simulink model "Cruise_Control_plant_model_with_continuous_controller"  (R2026a)
settings: Solver=VariableStepAuto  StopTime=inf
model workspace (MAT data in the model file):
  Crr = 0.015
  DragCoeff = 50
  MaxBrakeForce_N = 8000
  MaxEngineForce_N = 4000
  MaxVehicleSpeed_mps = 50
  MinCruiseSpd = 20
  Vehicle_mass_kg = 1000
  g = 9.81
libraries: slpidlib x1
settings Model: Creator=irfan  LastModifiedBy=irfan

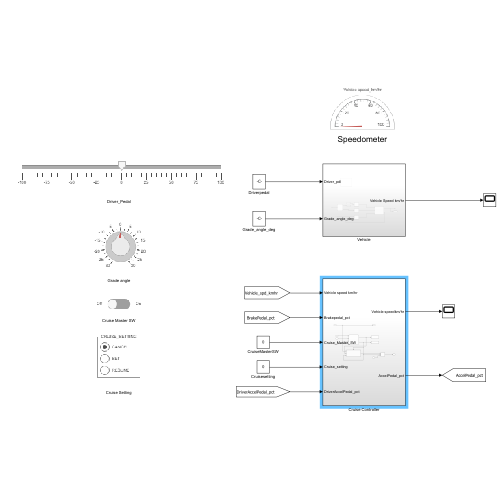
[thumbnail: Simulink's stored preview of the top-level diagram]
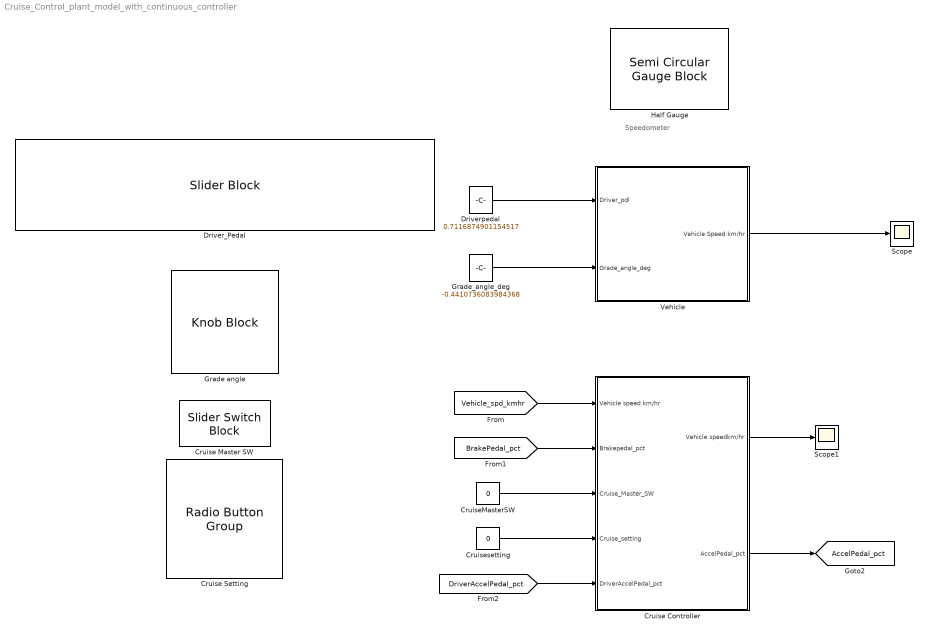
== system Cruise_Control_plant_model_with_continuous_controller ==
  note: Speedometer
  Cruise Controller : Subsystem
  Cruise Master SW : SliderSwitchBlock  LabelPosition=Hide
  Cruise Setting : RadioButtonGroup  LabelPosition=Hide  SelectedLabel=CANCEL  ButtonGroupName=CRUISE_SETTING
  CruiseMasterSW : Constant  Value=0
  Cruisesetting : Constant  Value=0
  Driver_Pedal : SliderBlock  LabelPosition=Hide  ScaleMin=-100  TickInterval=25
  Driverpedal : Constant  Value=0.7116874901154517
  Grade angle : KnobBlock  LabelPosition=Hide  ScaleMin=-30  ScaleMax=30  TickInterval=5
  Grade_angle_deg : Constant  Value=-0.4410736083984368
  Half Gauge : SemiCircularGaugeBlock  FontColor=[0.0, 0.0, 0.0]
  Scope : Scope
      settings: ActiveDisplayYMinimum=-1  ActiveDisplayYMaximum=1
  Scope1 : Scope
      settings: ActiveDisplayYMinimum=-1  ActiveDisplayYMaximum=1
  Vehicle : Subsystem
  tag scope: AccelPedal_pct=global
  wires:
  Vehicle/1(Vehicle Speed km/hr) -> Scope/1
  Driverpedal/1 -> Vehicle/1(Driver_pdl)
  Grade_angle_deg/1 -> Vehicle/2(Grade_angle_deg)
  [Vehicle_spd_kmhr] -> Cruise Controller/1(Vehicle speed km/hr)
  [BrakePedal_pct] -> Cruise Controller/2(Brakepedal_pct)
  Cruisesetting/1 -> Cruise Controller/4(Cruise_setting)
  CruiseMasterSW/1 -> Cruise Controller/3(Cruise_Master_SW)
  [DriverAccelPedal_pct] -> Cruise Controller/5(DriverAccelPedal_pct)
  Cruise Controller/2(AccelPedal_pct) -> [AccelPedal_pct]
  Cruise Controller/1(Vehicle speedkm/hr) -> Scope1/1

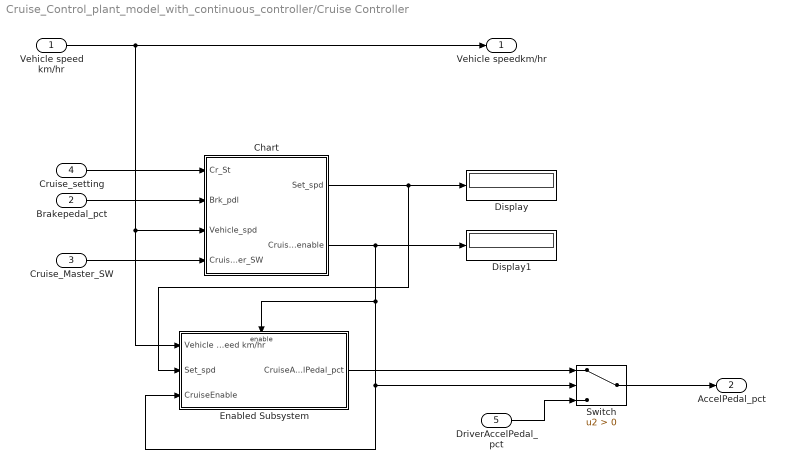
== system Cruise_Control_plant_model_with_continuous_controller/Cruise Controller ==
  Vehicle speed km/hr : Inport
  Brakepedal_pct : Inport  Port=2
  Cruise_Master_SW : Inport  Port=3
  Cruise_setting : Inport  Port=4
  DriverAccelPedal_pct : Inport  Port=5
  Chart : Stateflow chart  TreatAsAtomicUnit=on
  Display : Display
  Display1 : Display
  Enabled Subsystem : Subsystem  TreatAsAtomicUnit=on
  Switch : Switch  Criteria=u2 > Threshold  SaturateOnIntegerOverflow=off  InputSameDT=off
  Vehicle speedkm/hr : Outport
  AccelPedal_pct : Outport  Port=2
  wires:
  Cruise_setting/1 -> Chart/1(Cr_St)
  Brakepedal_pct/1 -> Chart/2(Brk_pdl)
  Vehicle speed km/hr/1 -> Vehicle speedkm/hr/1, Chart/3(Vehicle_spd), Enabled Subsystem/1(Vehicle speed km/hr)
  Chart/1(Set_spd) -> Enabled Subsystem/2(Set_spd), Display/1
  Chart/2(Cruise_enable) -> Display1/1, Enabled Subsystem/Enable, Enabled Subsystem/3(CruiseEnable), Switch/2
  Cruise_Master_SW/1 -> Chart/4(Cruise_Master_SW)
  Enabled Subsystem/1(CruiseAccelPedal_pct) -> Switch/1
  DriverAccelPedal_pct/1 -> Switch/3
  Switch/1 -> AccelPedal_pct/1

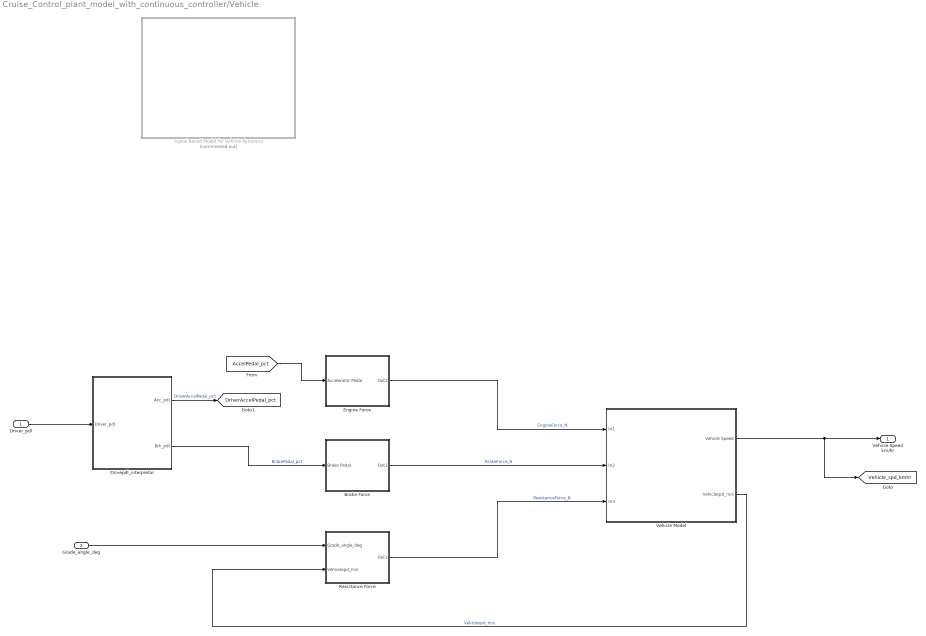
== system Cruise_Control_plant_model_with_continuous_controller/Vehicle ==
  Driver_pdl : Inport
  Grade_angle_deg : Inport  Port=2
  Brake Force : Subsystem
  Drivepdl_interpretor : Subsystem
  Engine Force : Subsystem
  Resistance Force : Subsystem
  Signal Based Model for Vehicle dynamics : Subsystem  Commented=on
  Vehicle Model : Subsystem
  Vehicle Speed km/hr : Outport
  tag scope: DriverAccelPedal_pct=global, Vehicle_spd_kmhr=global
  wires:
  Engine Force/1(Out1) -> Vehicle Model/1(In1)  "EngineForce_N"
  Brake Force/1(Out1) -> Vehicle Model/2(In2)  "BrakeForce_N"
  Drivepdl_interpretor/2(Brk_pdl) -> Brake Force/1(Brake Pedal)  "BrakePedal_pct"
  Resistance Force/1(Out1) -> Vehicle Model/3(In3)  "ResistanceForce_N"
  Vehicle Model/2(Vehiclespd_m/s) -> Resistance Force/2(Vehiclespd_m/s)  "Vehiclespd_m/s"
  Vehicle Model/1(Vehicle Speed) -> [Vehicle_spd_kmhr], Vehicle Speed km/hr/1
  Driver_pdl/1 -> Drivepdl_interpretor/1(Driver_pdl)
  Grade_angle_deg/1 -> Resistance Force/1(Grade_angle_deg)
  Drivepdl_interpretor/1(Acc_pdl) -> [DriverAccelPedal_pct]  "DriverAccelPedal_pct"
  [AccelPedal_pct] -> Engine Force/1(Accelerator Pedal)

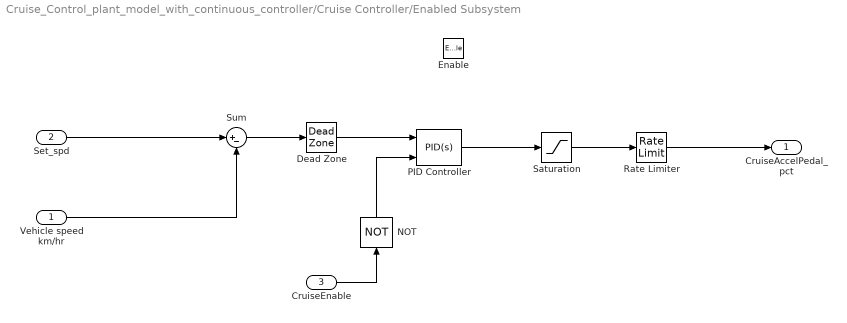
== system Cruise_Control_plant_model_with_continuous_controller/Cruise Controller/Enabled Subsystem ==
  Vehicle speed km/hr : Inport
  Set_spd : Inport  Port=2
  CruiseEnable : Inport  Port=3
  Enable : EnablePort  StatesWhenEnabling=reset
  Dead Zone : DeadZone
  NOT : Logic  Operator=NOT  IconShape=distinctive  AllPortsSameDT=off  OutDataTypeStr=boolean
  PID Controller : slpidlib/PID Controller  Controller=PID  Form=Parallel  TimeDomain=Continuous-time  UseExternalTs=off  SampleTime=-1  IntegratorMethod=Forward Euler  FilterMethod=Forward Euler  ControllerParametersSource=internal  P=1  I=0.5  UseKiTs=off  D=0  UseExternalDerivativeSource=off  N=100  UseFilter=on  TunerSelectOption=Transfer Function Based (PID Tuner App)  InitialConditionSource=internal  InitialConditionForIntegrator=0  InitialConditionForFilter=0  DifferentiatorICPrevScaledInput=0  ExternalReset=rising  TrackingMode=off  Kt=1  LimitOutput=on  SatLimitsSource=internal  UpperSaturationLimit=100  LowerSaturationLimit=0  LinearizeAsGain=on  AntiWindupMode=back-calculation  Kb=1  LimitIntegrator=off  UpperIntegratorSaturationLimit=inf  LowerIntegratorSaturationLimit=-inf  POutMin=[]  POutMax=[]  IOutMin=[]  IOutMax=[]  DOutMin=[]  DOutMax=[]  NOutMin=[]  NOutMax=[]  SumOutMin=[]  SumOutMax=[]  SaturationOutMin=[]  SaturationOutMax=[]  PParamMin=[]  PParamMax=[]  IParamMin=[]  IParamMax=[]  DParamMin=[]  DParamMax=[]  NParamMin=[]  NParamMax=[]  KbParamMin=[]  KbParamMax=[]  KtParamMin=[]  KtParamMax=[]  KbOutMin=[]  KbOutMax=[]  KtOutMin=[]  KtOutMax=[]  IntegratorOutMin=[]  IntegratorOutMax=[]  FilterOutMin=[]  FilterOutMax=[]  SumI1OutMin=[]  SumI1OutMax=[]  SumI2OutMin=[]  SumI2OutMax=[]  SumI3OutMin=[]  SumI3OutMax=[]  SumI4OutMin=[]  SumI4OutMax=[]  SumDOutMin=[]  SumDOutMax=[]  DifferentiatorOutMin=[]  DifferentiatorOutMax=[]  FilterDiffOutCoefMin=[]  FilterDiffOutCoefMax=[]  ReciprocalOutMin=[]  ReciprocalOutMax=[]  SumDenOutMin=[]  SumDenOutMax=[]  SumNumOutMin=[]  SumNumOutMax=[]  DivideOutMin=[]  DivideOutMax=[]  UdiffTsProdOutMin=[]  UdiffTsProdOutMax=[]  NTsProdOutMin=[]  NTsProdOutMax=[]  UintegralTsProdOutMin=[]  UintegralTsProdOutMax=[]  UngainTsProdOutMin=[]  UngainTsProdOutMax=[]  ClampingZeroOutDataTypeStr=Inherit: Inherit via back propagation  ClampingZeroOutMin=[]  ClampingZeroOutMax=[]  FilterDenConstantOutDataTypeStr=Inherit: Inherit via back propagation  FilterDenConstantOutMin=[]  FilterDenConstantOutMax=[]  PCopyOutDataTypeStr=Inherit: Inherit via back propagation  PCopyOutMin=[]  PCopyOutMax=[]  NCopyOutDataTypeStr=Inherit: Inherit via back propagation  NCopyOutMin=[]  NCopyOutMax=[]  IntegratorContinuousStateAttributes=''  IntegratorStateMustResolveToSignalObject=off  IntegratorRTWStateStorageClass=Auto  FilterContinuousStateAttributes=''  FilterStateMustResolveToSignalObject=off  FilterRTWStateStorageClass=Auto  ParallelPVariant=InternalParameters  IdealPVariant=Disabled  IVariant=InternalParameters  DVariant=InternalParameters  IntegratorVariant=Continuous  SatVariant=Enabled  AWVariant=BackCalculation  PCopyVariant=Disabled  TRVariant=Disabled  FdbkBlocksVariant=Forward  IdealPFdbkVariant=Disabled  SatFdbkVariant=Disabled  DerivativeFilterVariant=ContFilter  NVariant=InternalParameters  NCopyVariant=Disabled  FilterICVariant=InternalICsFilter  IntegratorICVariant=InternalICs  ExternalResetVariant=ExternalReset  TRSumVariant=Passthrough  SumFdbkVariant=Disabled  SumVariant=Sum_PID  TsampFilterVariant=InternalTs  TsampNgainVariant=Passthrough  TsampIntegralVariant=Disabled_SignalSpec  ExternalSaturationOutDataTypeStr=Inherit: Same as second input  DerivativeSourceVariant=ErrorSignal  PreIntVariant=InternalPreInt
  Rate Limiter : RateLimiter  RisingSlewLimit=25  FallingSlewLimit=-40  SampleTimeMode=inherited
  Saturation : Saturate  UpperLimit=100  LowerLimit=0
  Sum : Sum  Inputs=|+-
  CruiseAccelPedal_pct : Outport
  wires:
  Sum/1 -> Dead Zone/1
  Saturation/1 -> Rate Limiter/1
  CruiseEnable/1 -> NOT/1
  NOT/1 -> PID Controller/2
  Vehicle speed km/hr/1 -> Sum/2
  Set_spd/1 -> Sum/1
  PID Controller/1 -> Saturation/1
  Rate Limiter/1 -> CruiseAccelPedal_pct/1
  Dead Zone/1 -> PID Controller/1

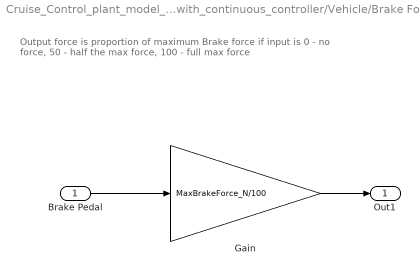
== system Cruise_Control_plant_model_with_continuous_controller/Vehicle/Brake Force ==
  note: Output force is proportion of maximum Brake force
      | if input is 0 - no force, 50 - half the max force, 100 - full max force
  Brake Pedal : Inport
  Gain : Gain  Gain=MaxBrakeForce_N/100
  Out1 : Outport
  wires:
  Brake Pedal/1 -> Gain/1
  Gain/1 -> Out1/1

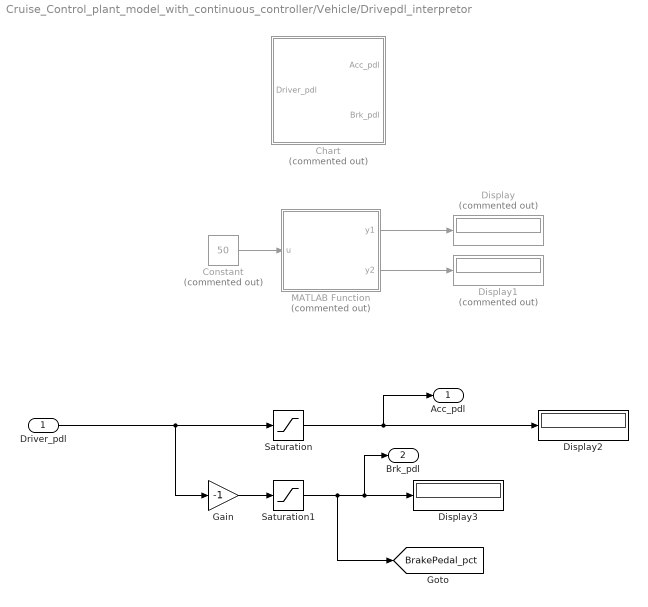
== system Cruise_Control_plant_model_with_continuous_controller/Vehicle/Drivepdl_interpretor ==
  Driver_pdl : Inport
  Chart : Stateflow chart  Commented=on  TreatAsAtomicUnit=on
  Constant : Constant  Commented=on  Value=50
  Display : Display  Commented=on
  Display1 : Display  Commented=on
  Display2 : Display
  Display3 : Display
  Gain : Gain  Gain=-1
  MATLAB Function : MATLAB Function  Commented=on  TreatAsAtomicUnit=on
  Saturation : Saturate  UpperLimit=100  LowerLimit=0
  Saturation1 : Saturate  UpperLimit=100  LowerLimit=0
  Acc_pdl : Outport
  Brk_pdl : Outport  Port=2
  tag scope: BrakePedal_pct=global
  wires:
  Constant/1 -> MATLAB Function/1(u)
  MATLAB Function/1(y1) -> Display/1
  MATLAB Function/2(y2) -> Display1/1
  Driver_pdl/1 -> Gain/1, Saturation/1
  Saturation/1 -> Acc_pdl/1, Display2/1
  Saturation1/1 -> [BrakePedal_pct], Brk_pdl/1, Display3/1
  Gain/1 -> Saturation1/1

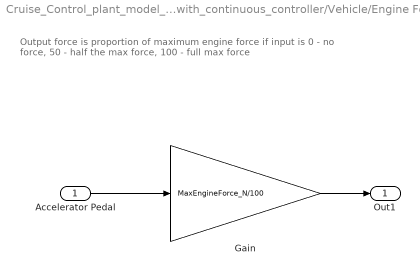
== system Cruise_Control_plant_model_with_continuous_controller/Vehicle/Engine Force ==
  note: Output force is proportion of maximum engine force
      | if input is 0 - no force, 50 - half the max force, 100 - full max force
  Accelerator Pedal : Inport
  Gain : Gain  Gain=MaxEngineForce_N/100
  Out1 : Outport
  wires:
  Accelerator Pedal/1 -> Gain/1
  Gain/1 -> Out1/1

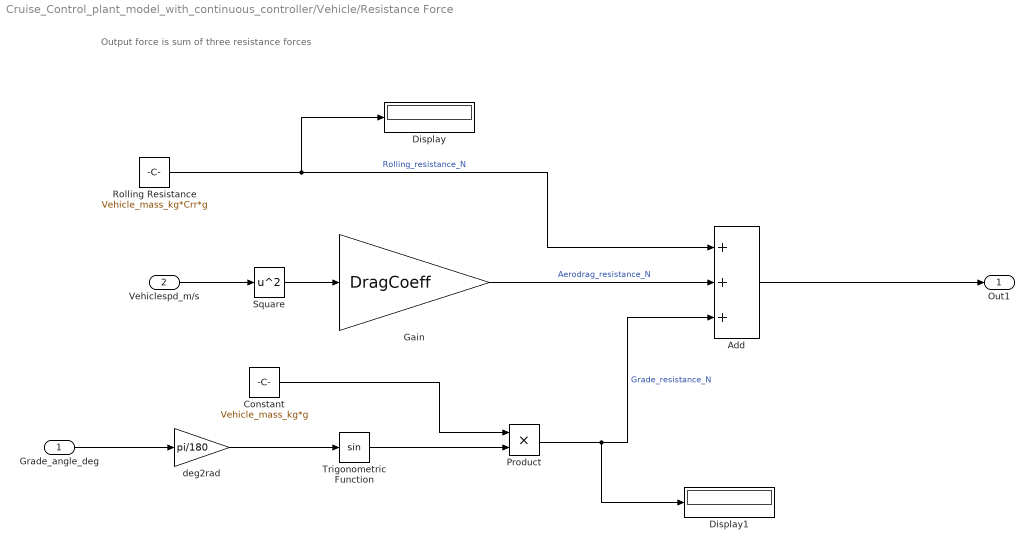
== system Cruise_Control_plant_model_with_continuous_controller/Vehicle/Resistance Force ==
  note: Output force is sum of three resistance forces
  Grade_angle_deg : Inport
  Vehiclespd_m/s : Inport  Port=2
  Add : Sum  Inputs=+++
  Constant : Constant  Value=Vehicle_mass_kg*g
  Display : Display
  Display1 : Display
  Gain : Gain  Gain=DragCoeff
  Product : Product
  Rolling Resistance : Constant  Value=Vehicle_mass_kg*Crr*g
  Square : Math  Operator=square
  Trigonometric Function : Trigonometry
  deg2rad : Gain  Gain=pi/180
  Out1 : Outport
  wires:
  Vehiclespd_m/s/1 -> Square/1
  Gain/1 -> Add/2  "Aerodrag_resistance_N"
  Rolling Resistance/1 -> Display/1, Add/1  "Rolling_resistance_N"
  Square/1 -> Gain/1
  Add/1 -> Out1/1
  Grade_angle_deg/1 -> deg2rad/1
  deg2rad/1 -> Trigonometric Function/1
  Trigonometric Function/1 -> Product/2
  Constant/1 -> Product/1
  Product/1 -> Display1/1, Add/3  "Grade_resistance_N"

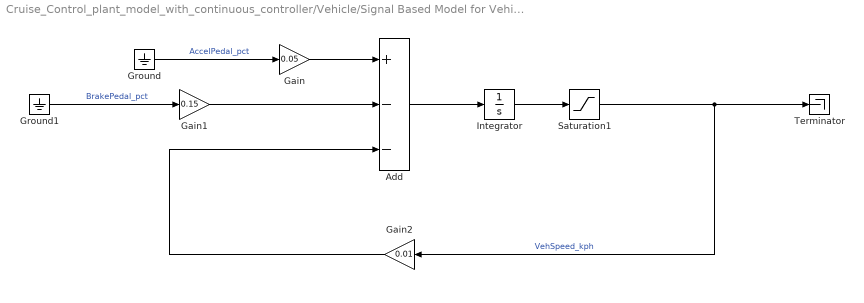
== system Cruise_Control_plant_model_with_continuous_controller/Vehicle/Signal Based Model for Vehicle dynamics ==
  Add : Sum  Inputs=+--
  Gain : Gain  Gain=0.05
  Gain1 : Gain  Gain=0.15
  Gain2 : Gain  Gain=0.01
  Ground : Ground
  Ground1 : Ground
  Integrator : Integrator
  Saturation1 : Saturate  UpperLimit=180  LowerLimit=0
  Terminator : Terminator
  wires:
  Ground1/1 -> Gain1/1  "BrakePedal_pct"
  Add/1 -> Integrator/1
  Gain/1 -> Add/1
  Gain2/1 -> Add/3
  Gain1/1 -> Add/2
  Saturation1/1 -> Terminator/1, Gain2/1  "VehSpeed_kph"
  Ground/1 -> Gain/1  "AccelPedal_pct"
  Integrator/1 -> Saturation1/1

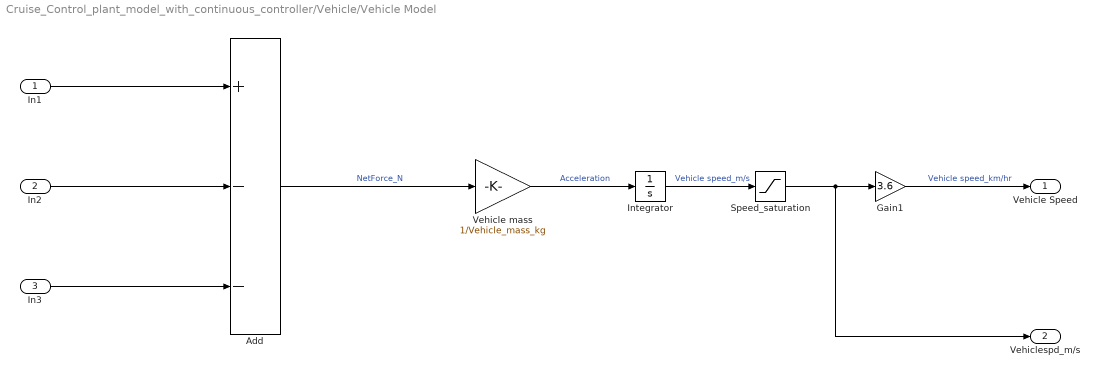
== system Cruise_Control_plant_model_with_continuous_controller/Vehicle/Vehicle Model ==
  In1 : Inport
  In2 : Inport  Port=2
  In3 : Inport  Port=3
  Add : Sum  Inputs=+--
  Gain1 : Gain  Gain=3.6
  Integrator : Integrator
  Speed_saturation : Saturate  UpperLimit=MaxVehicleSpeed_mps  LowerLimit=0
  Vehicle mass : Gain  Gain=1/Vehicle_mass_kg
  Vehicle Speed : Outport
  Vehiclespd_m/s : Outport  Port=2
  wires:
  In1/1 -> Add/1
  In2/1 -> Add/2
  In3/1 -> Add/3
  Add/1 -> Vehicle mass/1  "NetForce_N"
  Vehicle mass/1 -> Integrator/1  "Acceleration"
  Integrator/1 -> Speed_saturation/1  "Vehicle speed_m/s"
  Gain1/1 -> Vehicle Speed/1  "Vehicle speed_km/hr"
  Speed_saturation/1 -> Vehiclespd_m/s/1, Gain1/1

== stateflow chart Cruise_Control_plant_model_with_continuous_controller/Cruise Controller/Chart ==
  state READY
    entry:
    Set_spd = Vehicle_spd;
    Cruise_enable=0;
  state OFF
    during:
    Cruise_enable=0;
  state ACTIVE
    during:
    Cruise_enable=1;
  state STANDBY
    during:
    Cruise_enable=0;
  (default) -> OFF
  OFF -> READY : [Cruise_Master_SW==1 && Cr_St==1 && Vehicle_spd>MinCruiseSpd]
  READY -> (junction 19) [order 2]
  READY -> ACTIVE [order 1] : [true]
  (junction 19) -> OFF : [Cruise_Master_SW==0]
  ACTIVE -> (junction 19) [order 2]
  STANDBY -> (junction 19) [order 2]
  ACTIVE -> STANDBY [order 1] : [Cruise_Master_SW==1 && Cr_St==0 || Brk_pdl>0]
  STANDBY -> ACTIVE [order 1] : [Cruise_Master_SW==1 && Cr_St==2]
  data: Cr_St input; Brk_pdl input; Set_spd output; Cruise_enable output; Vehicle_spd input; MinCruiseSpd parameter; Cruise_Master_SW input

== matlab function Cruise_Control_plant_model_with_continuous_controller/Vehicle/Drivepdl_interpretor/MATLAB Function ==
  data: u input; y1 output; y2 output
function [y1, y2]= fcn(u)

y1=0;
y2=0;

if(u>0)
      y1=u;
      y2=0;
  
elseif (u<0)
       y1=0;
       y2=-u;
  
else
      y1=0;
      y2=0;
 
end

== stateflow chart Cruise_Control_plant_model_with_continuous_controller/Vehicle/Drivepdl_interpretor/Chart ==
  state Positive
    during:
    Acc_pdl=Driver_pdl;
    Brk_pdl=0;
  state Negative
    during:
    Brk_pdl= -1*Driver_pdl;
    Acc_pdl=0;
  state Zero
    during:
    Acc_pdl=0;
    Brk_pdl=0;
  (default) -> Positive
  Negative -> Positive [order 1] : [(Driver_pdl>0)]
  Positive -> Negative [order 1] : [(Driver_pdl<0)]
  Zero -> Positive [order 1] : [[(Driver_pdl>0)]]
  Positive -> Zero [order 2] : [[(Driver_pdl==0)]]
  Negative -> Zero [order 2] : [[[(Driver_pdl==0)]]]
  Zero -> Negative [order 2] : [[(Driver_pdl<0)]]
  data: Driver_pdl input; Acc_pdl output; Brk_pdl output
